simulink model "LLC_26"  (R2022b)
settings: Solver=VariableStepAuto  StartTime=0.0  StopTime=.01  RelTol=1e-3
values from neighbouring files (symbols this model uses):
  tsample_Controller = 20e-6    (= 2e-05)    [LLC_Parameter.m]
  Vref = 500    [LLC_Parameter.m]
undefined symbols (not defined in the file or in its folder): Iref
libraries: fl_lib x137, ee_lib x83, nesl_utility x63, slpidlib x7, slctrlblks x1
(part 1 of 5)
settings Model: Creator=HW-2  LastModifiedBy=Lenovo
settings DebuggingCC: UnconnectedInputMsg=warning  UnconnectedOutputMsg=warning  UnconnectedLineMsg=warning
settings ModelReferenceCC: EnableRefExpFcnMdlSchedulingChecks=on
settings RTWCC: DLArmComputeVersion=19.05

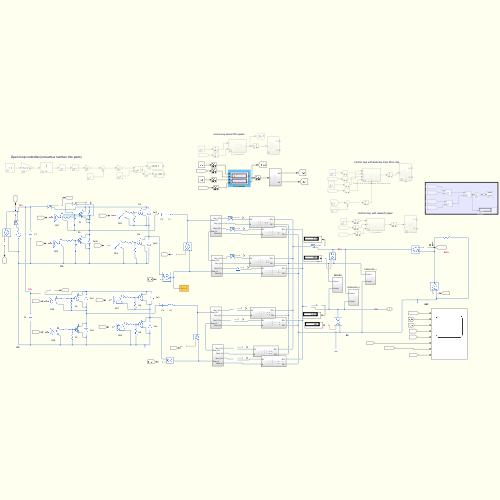
[thumbnail: Simulink's stored preview of the top-level diagram]
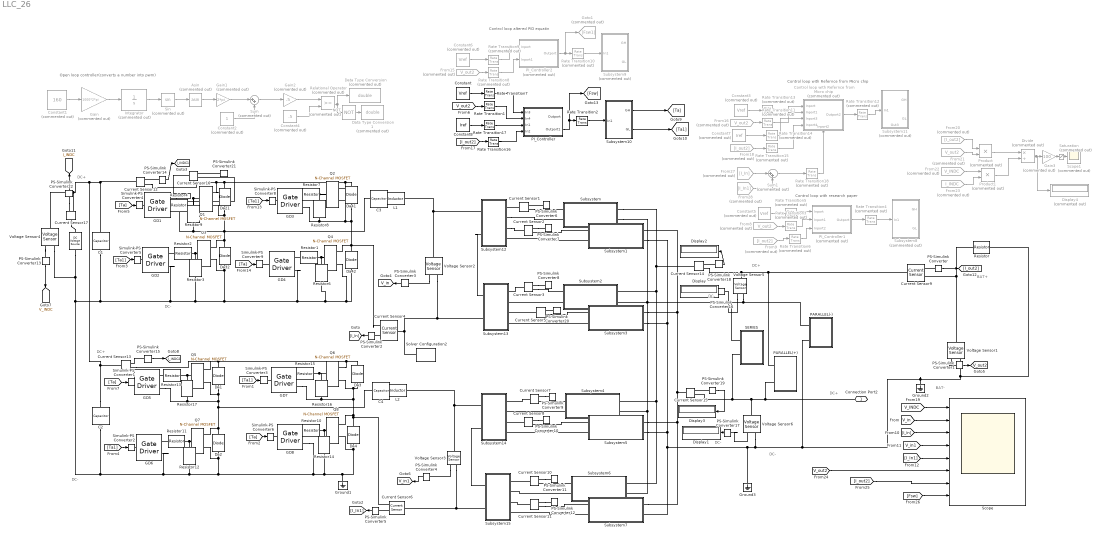
== system LLC_26 ==
  note: Open loop controller(converts a number into pwm)
  note: Control loop altered PID equatin
  note: DC+
  note: Control loop with Refernce from Micro chip
  note: DC-
  note: DC+
  note: Control loop with research paper
  note: BAT-
  note: DC-
  note: DC+
  note: DC-
  note: DC-
  note: DC-
  note: DC+
  note: BAT+
  " " : ee_lib/Additional Components/SPICE Sources/DC Voltage Source  DC=V_INDC V
  Asin : Trigonometry  Commented=on  Operator=asin
  C1 : fl_lib/Electrical/Electrical Elements/Capacitor  c=5e-6 F  r=5e-3 Ohm  g=0 1/Ohm  i_specify=off  i_priority=None  i=0 A  i_nominal_specify=off  i_nominal_unit=A  i_nominal_value=1  v_specify=off  v_priority=None  v=V_INDC V  v_nominal_specify=off  v_nominal_unit=V  v_nominal_value=1  vc_specify=on  vc_priority=High  vc=V_INDC V  vc_nominal_specify=off  vc_nominal_unit=V  vc_nominal_value=1
  C2 : fl_lib/Electrical/Electrical Elements/Capacitor  c=5e-6 F  r=5e-3 Ohm  g=0 1/Ohm  i_specify=off  i_priority=None  i=0 A  i_nominal_specify=off  i_nominal_unit=A  i_nominal_value=1  v_specify=off  v_priority=None  v=V_INDC V  v_nominal_specify=off  v_nominal_unit=V  v_nominal_value=1  vc_specify=on  vc_priority=High  vc=V_INDC V  vc_nominal_specify=off  vc_nominal_unit=V  vc_nominal_value=1
  C3 : fl_lib/Electrical/Electrical Elements/Capacitor  c=Cr F  r=0 Ohm  g=0 1/Ohm  i_specify=off  i_priority=None  i=0 A  i_nominal_specify=off  i_nominal_unit=A  i_nominal_value=1  v_specify=off  v_priority=None  v=0 V  v_nominal_specify=off  v_nominal_unit=V  v_nominal_value=1  vc_specify=off  vc_priority=High  vc=0 V  vc_nominal_specify=off  vc_nominal_unit=V  vc_nominal_value=1
  C4 : fl_lib/Electrical/Electrical Elements/Capacitor  c=Cr F  r=0 Ohm  g=0 1/Ohm  i_specify=off  i_priority=None  i=0 A  i_nominal_specify=off  i_nominal_unit=A  i_nominal_value=1  v_specify=off  v_priority=None  v=0 V  v_nominal_specify=off  v_nominal_unit=V  v_nominal_value=1  vc_specify=off  vc_priority=High  vc=0 V  vc_nominal_specify=off  vc_nominal_unit=V  vc_nominal_value=1
  Constant : Constant  Value=Vref
  Constant1 : Constant  Commented=on  Value=160
  Constant2 : Constant  Commented=on
  Constant3 : Constant  Commented=on  Value=Vref
  Constant4 : Constant  Commented=on  Value=.5
  Constant5 : Constant  Commented=on  Value=Vref
  Constant6 : Constant  Commented=on  Value=Vref
  Constant7 : Constant  Commented=on  Value=Iref
  Constant8 : Constant  Value=Iref
  Control loop with Refernce from Micro chip : Subsystem  Commented=on
      settings: PortSchema="{\"entries\":[{\"content\":{\"sides\":[{\"content\":{\"connectorIds\":[\"In1\",\"In2\",\"In3\",\"In4\"]},\"type\":\"ConnectorPlacement.EquallySpacedRectSide\",\"uuid\":\"8758e69c-c30c-4bdc-ab0d-0d062e0b37b7\"},{\"content\":{\"connectorIds\":[\"Out1\"],\"side\":\"RIGHT\"},\"type\":\"ConnectorPlacement.EquallySpacedRectSide\",\"uuid\":\"dabc2d05-f5c7-433d-b7be-f864c65222bf\"},{\"content\":{\"connectorIds\":[],\"side\":\"TOP\"},\"type\":\"ConnectorPlacement.EquallySpacedRectSide\",\"uuid\":\"e73110cd-836c-4139-8386-715c0e6c244a\"},{\"content\":{\"connectorIds\":[\"In5\"],\"side\":\"BOTTOM\"},\"type\":\"ConnectorPlacement.EquallySpacedRectSide\",\"uuid\":\"c3cb1167-cec3-47ee-be27-ca9bcd7e70cc\"}]},\"type\":\"ConnectorPlacement.EquallySpacedConnector\",\"uuid\":\"6b131b25-3151-447e-9ac8-8b0f0e72c048\"}],\"packageUris\":[\"http://schema.mathworks.com/mf0/Connector/R2020b\"],\"version\":\"1.0\"}"
  Current Sensor{1..17} (17 alike) : fl_lib/Electrical/Electrical Sensors/Current Sensor
  Da{1..4,21,32,41..42} (8 alike) : ee_lib/Semiconductors & Converters/Diode  ModelType=ee.enum.diode.modelType.pwl  TableType=ee.enum.diode.tableType.IfMat  IfMat=[.07, .12, .19, 1.75, 4.24, 7.32, 11.2; .16, .3, .72, 2.14, 4.02, 6.35, 9.12] A  VfMat=[.9, 1.15, 1.25, 1.5, 1.75, 2.17, 2.6, 2.85; .58, .68, .75, 1.1, 1.38, 1.77, 2.27, 2.7] V  TjVec=[25, 125] degC  VfVec=[.5, .7, .9, 1.3, 1.7, 2.1, 2.5] V  IfVec=[.1, .2, .5, 1, 2, 4, 7, 10] A  Vf=Vf V  Ron=Ron Ohm  Goff=1e-8 1/Ohm  prmExp=ee.enum.diode.expParam.useTwo  I12=[.0137, .545] A  V12=[.6, .7] V  RS=0 Ohm  Tmeas=25 degC  IS=1e-12 A  ec=1  I1=0.0137 A  V1=0.6 V  N_series=1  N_parallel=1  Rz=0.3 Ohm  BV=inf V  C_param=ee.enum.diode.capParam.fixed  CJ=0 pF  CJ0=5 pF  Vvec=[.1, 10, 100] V  Cvec=[3.5, 1, .4] pF  VJ=1 V  Mgrad=0.5  FC=0.5  Q_param=ee.enum.diode.recoveryParam.off  iRM=-7.15 A  iF=4 A  didt=-750 A/us  trr_factor=3  trr=115 ns  Qrr=1500 s*uA  Vr=-600 V  Ls=150 nH  Erec=0.03 J  TT=50 ns  tau=100 ns  T_param=ee.enum.diode.temperatureParam.off  Tdevice=25 degC  I1_T2=0.245 A  V1_T2=0.5 V  IS_T2=1.25e-7 A  Tmeas2=125 degC  XTI_param=ee.enum.diode.xtiParam.pn  XTI=3  EG_param=ee.enum.diode.egapParam.material_si  EG=1.11 eV  dBVdT=0 V/K  enable_faults=simscape.enum.onoff.off  fault_action=simscape.enum.assert.action.none  fault_types=ee.enum.diode.faults.open  tau_fault=1e-3 s  IfMat_faulted=[.07, .12, .19, 1.75, 4.24, 7.32, 11.2; .16, .3, .72, 2.14, 4.02, 6.35, 9.12] A  VfMat_faulted=[.9, 1.15, 1.25, 1.5, 1.75, 2.17, 2.6, 2.85; .58, .68, .75, 1.1, 1.38, 1.77, 2.27, 2.7] V  VfVec_faulted=[.5, .7, .9, 1.3, 1.7, 2.1, 2.5] V  IfVec_faulted=[.1, .2, .5, 1, 2, 4, 7, 10] A  Ropen_faulted=1000 Ohm  Gshort_faulted=1000 1/Ohm  Vf_faulted=0.6 V  Ron_faulted=0.3 Ohm  Goff_faulted=1e-8 S  I12_faulted=[.0137, .545] A  V12_faulted=[.6, .7] V  IS_faulted=1e-12 A  ec_faulted=1  I1_faulted=0.0137 A  V1_faulted=0.6 V  RS_faulted=0 Ohm  Rz_faulted=0.3 Ohm  BV_faulted=inf V  Cscale_faulted=100  enable_temporal_fault=simscape.enum.onoff.off  t_fault=inf s  enable_behavioral_fault=simscape.enum.onoff.off  max_permissible_voltage=inf V  n_fail_on_voltage=1  max_permissible_current=inf A  t_fail_on_current=1 s  max_permissible_dVdt=inf V/s  enable_fault_input=simscape.enum.onoff.off  i_specify=off  i_priority=None  i=0 A  i_nominal_specify=off  i_nominal_unit=A  i_nominal_value=1  v_specify=off  v_priority=None  v=0 V  v_nominal_specify=off  v_nominal_unit=V  v_nominal_value=1  v_capacitor_specify=off  v_capacitor_priority=None  v_capacitor=0 V  v_capacitor_nominal_specify=off  v_capacitor_nominal_unit=V  v_capacitor_nominal_value=1  i_diode_specify=off  i_diode_priority=None  i_diode=0 A  i_diode_nominal_specify=off  i_diode_nominal_unit=A  i_diode_nominal_value=1  v_diode_specify=off  v_diode_priority=None  v_diode=0 V  v_diode_nominal_specify=off  v_diode_nominal_unit=V  v_diode_nominal_value=1  i_capacitor_specify=off  i_capacitor_priority=None  i_capacitor=0 A  i_capacitor_nominal_specify=off  i_capacitor_nominal_unit=A  i_capacitor_nominal_value=1  power_dissipated_specify=off  power_dissipated_priority=None  power_dissipated=0 W  power_dissipated_nominal_specify=off  power_dissipated_nominal_unit=W  power_dissipated_nominal_value=1  fidelity_level=ee.enum.diode.fidelity.includeChargeDyn  rec_loss_model=ee.enum.diode.reverseRecoveryModel.fixed  ErecVal=0 J  ErecMat=zeros(2, 3) J  TjrecVec=[298.15, 398.15] K  IfrecVec=[.1, 1, 10] A  VrecVal=10 V  tFilter=1 / 1000 / 100 s  max_permissible_temperature=inf K  t_fail_on_temperature=1 s  thermal_network_parameterization=ee.enum.thermalNetworkTopology.junctionCase  Rth=[0, 10] K/W  Rth_Cauer=[1, 3, 10] K/W  Rth_Foster=[4, 6] K/W  thermal_mass_parameterization=ee.enum.thermalNetwork.timeconstant  thermal_mass=[0, 1] J/K  thermal_mass_Cauer=[.1, .3, 1] J/K  thermal_mass_Foster=[1.5, 3] J/K  thermal_time_constant=[0, 10] s  thermal_time_constant_Cauer=[1, 3, 10] s  thermal_time_constant_Foster=[6, 18] s  thermal_mass_initial_temperatures=[25, 25] degC  thermal_mass_initial_temperatures_Cauer=[25, 25, 25] degC  junction_thermal_mass=0.01 J/K  Tvec_initial_Foster=[25, 25, 25, 25] degC  no_thermal_network=0  junction_temperature_specify=off  junction_temperature_priority=None  junction_temperature=25 degC  junction_temperature_nominal_specify=off  junction_temperature_nominal_unit=degC  junction_temperature_nominal_value=1
  Data Type Conversion : DataTypeConversion  Commented=on  OutDataTypeStr=double  SaturateOnIntegerOverflow=off  RndMeth=Floor
  Data Type Conversion1 : DataTypeConversion  Commented=on  OutDataTypeStr=double  SaturateOnIntegerOverflow=off  RndMeth=Floor
  Display{,1..3} (4 alike) : Display
  Display4 : Display  Commented=on
  Divide : Product  Commented=on  Inputs=*/
  From{8,15..16,21} (4 alike) : From  Commented=on  GotoTag=V_out2  TagVisibility=global
  From18 : From  Commented=on  GotoTag=I_out2
  From20 : From  Commented=on  GotoTag=I_out2
  From22 : From  Commented=on  GotoTag=V_INDC  TagVisibility=global
  From23 : From  Commented=on  GotoTag=I_INDC  TagVisibility=global
  From27 : From  Commented=on  GotoTag=I_In
  From28 : From  Commented=on  GotoTag=I_In1
  From9 : From  Commented=on  GotoTag=I_out2
  GD{1..8} (8 alike) : ee_lib/Semiconductors & Converters/Gate Driver  uHighValue=0.7  uLowValue=0.3  vHigh=18 V  vLow=-3 V  tHigh=50 ns  tLow=50 ns  parameterization=1  rHigh=2 Ohm  rLow=2 Ohm  tRise=20 ns  tFall=20 ns  cLoad=10 nF  enable_faults=0  t_fault=1 s  fault_type=1  ZonTime_specify=off  ZonTime_priority=None  ZonTime=0 s  ZoffTime_specify=off  ZoffTime_priority=None  ZoffTime=0 s  uHigh=2.0 V  uLow=0.8 V
      settings: InternalSimscapePortConfiguration="{\"Bottom\":[],\"Left\":[{\"id\":\"u\",\"label\":\"u\",\"type\":\"input\"}],\"Right\":[{\"id\":\"G\",\"label\":\"G\",\"type\":\"foundation.electrical.electrical\"},{\"id\":\"S\",\"label\":\"S\",\"type\":\"foundation.electrical.electrical\"}],\"Top\":[]}"
  Gain : Gain  Commented=on  Gain=1000*2*pi
  Gain1 : Gain  Commented=on  Gain=2*pi
  Gain2 : Gain  Commented=on  Gain=.5
  Gain3 : Gain  Commented=on  Gain=100
  Goto1 : Goto  Commented=on  GotoTag=Fsw1
  Ground1 : fl_lib/Electrical/Electrical Elements/Electrical Reference
  Ground2 : fl_lib/Electrical/Electrical Elements/Electrical Reference
  Ground3 : fl_lib/Electrical/Electrical Elements/Electrical Reference
  Integrator : Integrator  Commented=on
  L1 : fl_lib/Electrical/Electrical Elements/Inductor  l=Lr H  r=0 Ohm  g=0 1/Ohm  i_specify=off  i_priority=None  i=0 A  i_nominal_specify=off  i_nominal_unit=A  i_nominal_value=1  v_specify=off  v_priority=None  v=0 V  v_nominal_specify=off  v_nominal_unit=V  v_nominal_value=1  i_L_specify=off  i_L_priority=High  i_L=0 A  i_L_nominal_specify=off  i_L_nominal_unit=A  i_L_nominal_value=1
  L2 : fl_lib/Electrical/Electrical Elements/Inductor  l=Lr H  r=0 Ohm  g=0 1/Ohm  i_specify=off  i_priority=None  i=0 A  i_nominal_specify=off  i_nominal_unit=A  i_nominal_value=1  v_specify=off  v_priority=None  v=0 V  v_nominal_specify=off  v_nominal_unit=V  v_nominal_value=1  i_L_specify=off  i_L_priority=High  i_L=0 A  i_L_nominal_specify=off  i_L_nominal_unit=A  i_L_nominal_value=1
  NOT : Logic  Commented=on  Operator=NOT  IconShape=distinctive  AllPortsSameDT=off  OutDataTypeStr=boolean
  PARALLEL(+) : Subsystem
  PARALLEL(-) : Subsystem
  PI_Controller : Subsystem
  PI_Controller1 : Subsystem  Commented=on
  PI_Controller2 : Subsystem  Commented=on
  PS-Simulink Converter{,1..22} (23 alike) : nesl_utility/PS-Simulink Converter  PhysicalDomain=network_engine_domain  SubClassName=ps_output  LeftPortType=input  RightPortType=output  PseudoPeriodic=off  Frequencies=[]  VectorFormat=1-D array  Unit=inherit  AffineConversion=off
  Product : Product  Commented=on
  Product1 : Product  Commented=on
  Q{1,3..8} (7 alike) : ee_lib/Semiconductors & Converters/N-Channel MOSFET  paramTerminal=ee.enum.mosfet.numberOfTerminals.three  parameterization=ee.enum.mosfet.parameterization.datasheet  Beta=5.0 A/V^2  Rds=0.042 Ohm  Id=100 A  Vgs=20 V  Vth=3.8 V  Vth0=2.8 V  lam=0 1/V  gamma_vth=0.5 V^0.50000  phib=0.5 V  Vth1=4 V  Vbs1=-1 V  Vth2=5 V  Vbs2=-2 V  Tmeas=125 degC  Vgs_vec=[-.5, 2, 3, 4, 5] V  Vds_vec=[0, 2, 4, 8, 12, 16, 20] V  Vbs_vec=[0, -4, -6, -12] V  T_vec=[25, 125] degC  Vth_vec=[.4, 1.2, 1.4, 1.45] V  Vth_mat=[.4, .35; 1.2, 1.15; 1.4, 1.35; 1.45, 1.4] V  Ids_mat=[0, 0, 0, 0, 0, 0, 0; 0, .003, .0038, .0043, .0046, .0048, .0049; 0, .0055, .008, .009, .0095, .01, .0101; 0, .0115, .016, .018, .019, .0195, .02; 0, .0152, .0225, .0265, .028, .0295, .03] A  Ids_mat0=[0, 0, 0, 0, 0, 0, 0; 0, .003, .0038, .0043, .0046, .0048, .0049; 0, .0055, .008, .009, .0095, .01, .0101; 0, .0115, .016, .018, .019, .0195, .02; 0, .0152, .0225, .0265, .028, .0295, .03] A  Ids_mat_3D=zeros(5, 7, 2) A  Ids_mat_3D0=zeros(5, 7, 2) A  IV_table_symmetry=ee.enum.mosfet.symmetricNIV.no  RS=1e-3 Ohm  RD=0.1e-3 Ohm  RB=0.001 Ohm  C_param=ee.enum.mosfet.capacitanceParam.fixedciss  C_GS=270 pF  C_GD=80 pF  C_GB=0 pF  C_DS=0 pF  C_iss=2320 pF  C_rss=9 pF  C_oss=111 pF  C_iss_vec=[720, 700, 590, 470, 390, 310] pF  C_rss_vec=[450, 400, 300, 190, 95, 55] pF  C_oss_vec=[900, 810, 690, 420, 270, 170] pF  C_GS_vec=[270, 300, 290, 280, 295, 255] pF  C_GD_vec=[450, 400, 300, 190, 95, 55] pF  C_GB_vec=[270, 300, 290, 280, 295, 255] pF  C_Vgs_vec=0 V  C_DS_vec=[450, 410, 390, 230, 175, 115] pF  C_Vds_vec=[.1, .3, 1, 3, 10, 30] V  V_GS_for_cap_data=0 V  charge_linearity_param=ee.enum.mosfet.cgdLinearity.constant  C_OX=200 pF  V_C_OX=-0.5 V  charge_linearity_param_vgb=ee.enum.mosfet.cgbLinearity.instantly  charge_linearity_param_with_vgb=ee.enum.mosfet.cgbLinearityWithSeparateCgb.instantly  Di_param=ee.enum.mosfet.diodeParam.no  IsDiode=0 A  Vbi=0.6 V  n=1  Cj0Diode=0 pF  TT=50e-9 s  Tmeas_dio=25 degC  TableTypeNoT=ee.enum.mosfet.tableType.IfMat  TableType=ee.enum.diode.tableType.IfMat  IfVec=[.07, .12, .19, 1.75, 4.24, 7.32, 11.2] A  IfMat=[.07, .12, .19, 1.75, 4.24, 7.32, 11.2; .16, .3, .72, 2.14, 4.02, 6.35, 9.12] A  VfVecV=[.9, 1.15, 1.25, 1.5, 1.75, 2.17, 2.6, 2.85] V  VfMatV=[.9, 1.15, 1.25, 1.5, 1.75, 2.17, 2.6, 2.85; .58, .68, .75, 1.1, 1.38, 1.77, 2.27, 2.7] V  TjVec=[25, 125] degC  VfVec=[.5, .7, .9, 1.3, 1.7, 2.1, 2.5] V  IfVecV=[.1, .2, .5, 1, 2, 4, 7, 10] A  prmDatasheet=ee.enum.temperatureParameterization.none  prmEquCoeff=ee.enum.temperatureParameterization.none  dVth_dT=-6 mV/K  dVth0_dT=-6 mV/K  Rds_T2=0.037 Ohm  BEXDatasheet=-1.5  BEXEquCoeff=-1.5  etaisDatasheet=3  etaisEquCoeff=3  Tmeas2=125 degC  etaisTabulated=3  TdeviceDatasheet=25 degC  TdeviceEquCoeff=25 degC  TdeviceTabulated=25 degC  enable_faults=simscape.enum.onoff.off  fault_trigger=ee.enum.faults.faultTrigger.temporal  t_fault=inf s  max_permissible_Vgs=inf V  max_permissible_Vds=inf V  max_permissible_Vdb=inf V  max_permissible_Ids=inf A  t_fail_on_Ids=1 s  max_permissible_Idiode=inf A  t_fail_on_Idiode=1 s  max_permissible_dVdt=inf V/s  tau_fault=1e-3 s  fault_types=ee.enum.mosfet.faults.open  fault_types_4T=ee.enum.mosfet.faultsFourTerminals.open  RG_open=1e6 Ohm  RD_open=1000 Ohm  RS_open=1000 Ohm  RB_open=1000 Ohm  GDS_short=1000 1/Ohm  GDB_short=1000 1/Ohm  GSB_short=1000 1/Ohm  location_GOS=0  G_GOS=1000 1/Ohm  D_GOS=ee.enum.include.no  Is_GOS=0 A  Vbi_GOS=0.6 V  n_GOS=1  Cj0_GOS=0 pF  TT_GOS=50e-9 s  Beta_scale=100  dVth_faulted=0 V  lam_faulted=0 1/V  gamma_scale=100  dPhib_faulted=0 V  Vgs_vec_faulted=[-.5, 2, 3, 4, 5] V  Vds_vec_faulted=[0, 2, 4, 8, 12, 16, 20] V  Vbs_vec_faulted=[0, -4, -6, -12] V  Vth_vec_faulted=[.4, 1.2, 1.4, 1.45] V  Vth_mat_faulted=[.4, .35; 1.2, 1.15; 1.4, 1.35; 1.45, 1.4] V  Ids_mat_faulted=[0, 0, 0, 0, 0, 0, 0; 0, .003, .0038, .0043, .0046, .0048, .0049; 0, .0055, .008, .009, .0095, .01, .0101; 0, .0115, .016, .018, .019, .0195, .02; 0, .0152, .0225, .0265, .028, .0295, .03] A  Ids_mat0_faulted=[0, 0, 0, 0, 0, 0, 0; 0, .003, .0038, .0043, .0046, .0048, .0049; 0, .0055, .008, .009, .0095, .01, .0101; 0, .0115, .016, .018, .019, .0195, .02; 0, .0152, .0225, .0265, .028, .0295, .03] A  Ids_mat_3D_faulted=zeros(5, 7, 2) A  Ids_mat_3D0_faulted=zeros(5, 7, 2) A  RS_faulted=0.0001 Ohm  RD_faulted=0.01 Ohm  RB_faulted=0.001 Ohm  IsDiode_faulted=0 A  Vbi_faulted=0.6 V  n_faulted=1  Cj0Diode_scale=100  TT_faulted=50e-9 s  IfVec_faulted=[.07, .12, .19, 1.75, 4.24, 7.32, 11.2] A  IfMat_faulted=[.07, .12, .19, 1.75, 4.24, 7.32, 11.2; .16, .3, .72, 2.14, 4.02, 6.35, 9.12] A  VfVecV_faulted=[.9, 1.15, 1.25, 1.5, 1.75, 2.17, 2.6, 2.85] V  VfMatV_faulted=[.9, 1.15, 1.25, 1.5, 1.75, 2.17, 2.6, 2.85; .58, .68, .75, 1.1, 1.38, 1.77, 2.27, 2.7] V  VfVec_faulted=[.5, .7, .9, 1.3, 1.7, 2.1, 2.5] V  IfVecV_faulted=[.1, .2, .5, 1, 2, 4, 7, 10] A  C_GS_scale=100  C_GD_scale=100  C_GB_scale=100  C_DS_scale=100  C_OX_scale=100  V_C_OX_faulted=-0.5 V  C_iss_vec_faulted=[720, 700, 590, 470, 390, 310] pF  C_rss_vec_faulted=[450, 400, 300, 190, 95, 55] pF  C_oss_vec_faulted=[900, 810, 690, 420, 270, 170] pF  C_GS_vec_faulted=[270, 300, 290, 280, 295, 255] pF  C_GD_vec_faulted=[450, 400, 300, 190, 95, 55] pF  C_GB_vec_faulted=[270, 300, 290, 280, 295, 255] pF  C_Vgs_vec_faulted=0 V  C_DS_vec_faulted=[450, 410, 390, 230, 175, 115] pF  C_Vds_vec_faulted=[.1, .3, 1, 3, 10, 30] V  V_GS_for_cap_data_faulted=0 V  i_g_specify=off  i_g_priority=None  i_g=0 A  i_g_nominal_specify=off  i_g_nominal_unit=A  i_g_nominal_value=1  i_d_specify=off  i_d_priority=None  i_d=0 A  i_d_nominal_specify=off  i_d_nominal_unit=A  i_d_nominal_value=1  i_b_specify=off  i_b_priority=None  i_b=0 A  i_b_nominal_specify=off  i_b_nominal_unit=A  i_b_nominal_value=1  voltage_gs_specify=off  voltage_gs_priority=None  voltage_gs=0 V  voltage_gs_nominal_specify=off  voltage_gs_nominal_unit=V  voltage_gs_nominal_value=1  voltage_ds_specify=off  voltage_ds_priority=None  voltage_ds=0 V  voltage_ds_nominal_specify=off  voltage_ds_nominal_unit=V  voltage_ds_nominal_value=1  voltage_bs_specify=off  voltage_bs_priority=None  voltage_bs=0 V  voltage_bs_nominal_specify=off  voltage_bs_nominal_unit=V  voltage_bs_nominal_value=1  v_Cgs_specify=off  v_Cgs_priority=High  v_Cgs=0 V  v_Cgs_nominal_specify=off  v_Cgs_nominal_unit=V  v_Cgs_nominal_value=1  v_Cds_specify=off  v_Cds_priority=High  v_Cds=0 V  v_Cds_nominal_specify=off  v_Cds_nominal_unit=V  v_Cds_nominal_value=1  v_Cbs_specify=off  v_Cbs_priority=High  v_Cbs=0 V  v_Cbs_nominal_specify=off  v_Cbs_nominal_unit=V  v_Cbs_nominal_value=1  thermal_network_parameterization=ee.enum.thermalNetworkTopology.junctionCase  Rth=[0, 10] K/W  Rth_Cauer=[1, 3, 10] K/W  Rth_Foster=[4, 6] K/W  thermal_mass_parameterization=ee.enum.thermalNetwork.timeconstant  thermal_mass=[0, 1] J/K  thermal_mass_Cauer=[.1, .3, 1] J/K  thermal_mass_Foster=[1.5, 3] J/K  thermal_time_constant=[0, 10] s  thermal_time_constant_Cauer=[1, 3, 10] s  thermal_time_constant_Foster=[6, 18] s  thermal_mass_initial_temperatures=[25, 25] degC  thermal_mass_initial_temperatures_Cauer=[25, 25, 25] degC  Tvec_initial_Foster=[25, 25, 25, 25] degC  max_permissible_temperature=inf K  t_fail_on_temperature=1 s  betaref=18 A/V^2  Vfbref=-1.1 V  gamma=3.5 V^(1/2)  phib2ref=1 V  thesatref=0.4 1/V  alpha=0  Vp=5e-2 V  thesrref=0 1/V  m=8  Tref=25 degC  Rsref=2e-3 Ohm  Rdref=0.17 Ohm  Rgref=8.4 Ohm  Rbref=2e-3 Ohm  Cox=1500 pF  Cgso=100 pF  Cgdo=14 pF  Isref=5.2e-13 A  Cj0=480 pF  Tprm=1  etabet=1.3  Stvfb=5e-4 V/K  Stphib=-8.5e-4 V/K  etasat=1.04  etasr=0.65  etar=0.95  etais=3  Tsim=25 degC  Ig_specify=off  Ig_priority=None  Ig=0 A  Ig_nominal_specify=off  Ig_nominal_unit=A  Ig_nominal_value=1  Ids_specify=off  Ids_priority=None  Ids=0 A  Ids_nominal_specify=off  Ids_nominal_unit=A  Ids_nominal_value=1  Ib_specify=off  Ib_priority=None  Ib=0 A  Ib_nominal_specify=off  Ib_nominal_unit=A  Ib_nominal_value=1  V_gs_specify=off  V_gs_priority=None  V_gs=0 V  V_gs_nominal_specify=off  V_gs_nominal_unit=V  V_gs_nominal_value=1  V_ds_specify=off  V_ds_priority=None  V_ds=0 V  V_ds_nominal_specify=off  V_ds_nominal_unit=V  V_ds_nominal_value=1  V_bs_specify=off  V_bs_priority=None  V_bs=0 V  V_bs_nominal_specify=off  V_bs_nominal_unit=V  V_bs_nominal_value=1  QGoverCox_specify=off  QGoverCox_priority=None  QGoverCox=0 V  QGoverCox_nominal_specify=off  QGoverCox_nominal_unit=V  QGoverCox_nominal_value=1  QDoverCox_specify=off  QDoverCox_priority=None  QDoverCox=0 V  QDoverCox_nominal_specify=off  QDoverCox_nominal_unit=V  QDoverCox_nominal_value=1  QBoverCox_specify=off  QBoverCox_priority=None  QBoverCox=0 V  QBoverCox_nominal_specify=off  QBoverCox_nominal_unit=V  QBoverCox_nominal_value=1  T0=[25, 25] degC  T0_Cauer=[25, 25, 25] degC
  "Q2 " : ee_lib/Semiconductors & Converters/N-Channel MOSFET  paramTerminal=ee.enum.mosfet.numberOfTerminals.three  parameterization=ee.enum.mosfet.parameterization.datasheet  Beta=5.0 A/V^2  Rds=0.042 Ohm  Id=100 A  Vgs=20 V  Vth=3.8 V  Vth0=2.8 V  lam=0 1/V  gamma_vth=0.5 V^0.50000  phib=0.5 V  Vth1=4 V  Vbs1=-1 V  Vth2=5 V  Vbs2=-2 V  Tmeas=125 degC  Vgs_vec=[-.5, 2, 3, 4, 5] V  Vds_vec=[0, 2, 4, 8, 12, 16, 20] V  Vbs_vec=[0, -4, -6, -12] V  T_vec=[25, 125] degC  Vth_vec=[.4, 1.2, 1.4, 1.45] V  Vth_mat=[.4, .35; 1.2, 1.15; 1.4, 1.35; 1.45, 1.4] V  Ids_mat=[0, 0, 0, 0, 0, 0, 0; 0, .003, .0038, .0043, .0046, .0048, .0049; 0, .0055, .008, .009, .0095, .01, .0101; 0, .0115, .016, .018, .019, .0195, .02; 0, .0152, .0225, .0265, .028, .0295, .03] A  Ids_mat0=[0, 0, 0, 0, 0, 0, 0; 0, .003, .0038, .0043, .0046, .0048, .0049; 0, .0055, .008, .009, .0095, .01, .0101; 0, .0115, .016, .018, .019, .0195, .02; 0, .0152, .0225, .0265, .028, .0295, .03] A  Ids_mat_3D=zeros(5, 7, 2) A  Ids_mat_3D0=zeros(5, 7, 2) A  IV_table_symmetry=ee.enum.mosfet.symmetricNIV.no  RS=1e-3 Ohm  RD=0.1e-3 Ohm  RB=0.001 Ohm  C_param=ee.enum.mosfet.capacitanceParam.fixedciss  C_GS=270 pF  C_GD=80 pF  C_GB=0 pF  C_DS=0 pF  C_iss=2320 pF  C_rss=9 pF  C_oss=111 pF  C_iss_vec=[720, 700, 590, 470, 390, 310] pF  C_rss_vec=[450, 400, 300, 190, 95, 55] pF  C_oss_vec=[900, 810, 690, 420, 270, 170] pF  C_GS_vec=[270, 300, 290, 280, 295, 255] pF  C_GD_vec=[450, 400, 300, 190, 95, 55] pF  C_GB_vec=[270, 300, 290, 280, 295, 255] pF  C_Vgs_vec=0 V  C_DS_vec=[450, 410, 390, 230, 175, 115] pF  C_Vds_vec=[.1, .3, 1, 3, 10, 30] V  V_GS_for_cap_data=0 V  charge_linearity_param=ee.enum.mosfet.cgdLinearity.constant  C_OX=200 pF  V_C_OX=-0.5 V  charge_linearity_param_vgb=ee.enum.mosfet.cgbLinearity.instantly  charge_linearity_param_with_vgb=ee.enum.mosfet.cgbLinearityWithSeparateCgb.instantly  Di_param=ee.enum.mosfet.diodeParam.no  IsDiode=0 A  Vbi=0.6 V  n=1  Cj0Diode=0 pF  TT=50e-9 s  Tmeas_dio=25 degC  TableTypeNoT=ee.enum.mosfet.tableType.IfMat  TableType=ee.enum.diode.tableType.IfMat  IfVec=[.07, .12, .19, 1.75, 4.24, 7.32, 11.2] A  IfMat=[.07, .12, .19, 1.75, 4.24, 7.32, 11.2; .16, .3, .72, 2.14, 4.02, 6.35, 9.12] A  VfVecV=[.9, 1.15, 1.25, 1.5, 1.75, 2.17, 2.6, 2.85] V  VfMatV=[.9, 1.15, 1.25, 1.5, 1.75, 2.17, 2.6, 2.85; .58, .68, .75, 1.1, 1.38, 1.77, 2.27, 2.7] V  TjVec=[25, 125] degC  VfVec=[.5, .7, .9, 1.3, 1.7, 2.1, 2.5] V  IfVecV=[.1, .2, .5, 1, 2, 4, 7, 10] A  prmDatasheet=ee.enum.temperatureParameterization.none  prmEquCoeff=ee.enum.temperatureParameterization.none  dVth_dT=-6 mV/K  dVth0_dT=-6 mV/K  Rds_T2=0.037 Ohm  BEXDatasheet=-1.5  BEXEquCoeff=-1.5  etaisDatasheet=3  etaisEquCoeff=3  Tmeas2=125 degC  etaisTabulated=3  TdeviceDatasheet=25 degC  TdeviceEquCoeff=25 degC  TdeviceTabulated=25 degC  enable_faults=simscape.enum.onoff.off  fault_trigger=ee.enum.faults.faultTrigger.temporal  t_fault=inf s  max_permissible_Vgs=inf V  max_permissible_Vds=inf V  max_permissible_Vdb=inf V  max_permissible_Ids=inf A  t_fail_on_Ids=1 s  max_permissible_Idiode=inf A  t_fail_on_Idiode=1 s  max_permissible_dVdt=inf V/s  tau_fault=1e-3 s  fault_types=ee.enum.mosfet.faults.open  fault_types_4T=ee.enum.mosfet.faultsFourTerminals.open  RG_open=1e6 Ohm  RD_open=1000 Ohm  RS_open=1000 Ohm  RB_open=1000 Ohm  GDS_short=1000 1/Ohm  GDB_short=1000 1/Ohm  GSB_short=1000 1/Ohm  location_GOS=0  G_GOS=1000 1/Ohm  D_GOS=ee.enum.include.no  Is_GOS=0 A  Vbi_GOS=0.6 V  n_GOS=1  Cj0_GOS=0 pF  TT_GOS=50e-9 s  Beta_scale=100  dVth_faulted=0 V  lam_faulted=0 1/V  gamma_scale=100  dPhib_faulted=0 V  Vgs_vec_faulted=[-.5, 2, 3, 4, 5] V  Vds_vec_faulted=[0, 2, 4, 8, 12, 16, 20] V  Vbs_vec_faulted=[0, -4, -6, -12] V  Vth_vec_faulted=[.4, 1.2, 1.4, 1.45] V  Vth_mat_faulted=[.4, .35; 1.2, 1.15; 1.4, 1.35; 1.45, 1.4] V  Ids_mat_faulted=[0, 0, 0, 0, 0, 0, 0; 0, .003, .0038, .0043, .0046, .0048, .0049; 0, .0055, .008, .009, .0095, .01, .0101; 0, .0115, .016, .018, .019, .0195, .02; 0, .0152, .0225, .0265, .028, .0295, .03] A  Ids_mat0_faulted=[0, 0, 0, 0, 0, 0, 0; 0, .003, .0038, .0043, .0046, .0048, .0049; 0, .0055, .008, .009, .0095, .01, .0101; 0, .0115, .016, .018, .019, .0195, .02; 0, .0152, .0225, .0265, .028, .0295, .03] A  Ids_mat_3D_faulted=zeros(5, 7, 2) A  Ids_mat_3D0_faulted=zeros(5, 7, 2) A  RS_faulted=0.0001 Ohm  RD_faulted=0.01 Ohm  RB_faulted=0.001 Ohm  IsDiode_faulted=0 A  Vbi_faulted=0.6 V  n_faulted=1  Cj0Diode_scale=100  TT_faulted=50e-9 s  IfVec_faulted=[.07, .12, .19, 1.75, 4.24, 7.32, 11.2] A  IfMat_faulted=[.07, .12, .19, 1.75, 4.24, 7.32, 11.2; .16, .3, .72, 2.14, 4.02, 6.35, 9.12] A  VfVecV_faulted=[.9, 1.15, 1.25, 1.5, 1.75, 2.17, 2.6, 2.85] V  VfMatV_faulted=[.9, 1.15, 1.25, 1.5, 1.75, 2.17, 2.6, 2.85; .58, .68, .75, 1.1, 1.38, 1.77, 2.27, 2.7] V  VfVec_faulted=[.5, .7, .9, 1.3, 1.7, 2.1, 2.5] V  IfVecV_faulted=[.1, .2, .5, 1, 2, 4, 7, 10] A  C_GS_scale=100  C_GD_scale=100  C_GB_scale=100  C_DS_scale=100  C_OX_scale=100  V_C_OX_faulted=-0.5 V  C_iss_vec_faulted=[720, 700, 590, 470, 390, 310] pF  C_rss_vec_faulted=[450, 400, 300, 190, 95, 55] pF  C_oss_vec_faulted=[900, 810, 690, 420, 270, 170] pF  C_GS_vec_faulted=[270, 300, 290, 280, 295, 255] pF  C_GD_vec_faulted=[450, 400, 300, 190, 95, 55] pF  C_GB_vec_faulted=[270, 300, 290, 280, 295, 255] pF  C_Vgs_vec_faulted=0 V  C_DS_vec_faulted=[450, 410, 390, 230, 175, 115] pF  C_Vds_vec_faulted=[.1, .3, 1, 3, 10, 30] V  V_GS_for_cap_data_faulted=0 V  i_g_specify=off  i_g_priority=None  i_g=0 A  i_g_nominal_specify=off  i_g_nominal_unit=A  i_g_nominal_value=1  i_d_specify=off  i_d_priority=None  i_d=0 A  i_d_nominal_specify=off  i_d_nominal_unit=A  i_d_nominal_value=1  i_b_specify=off  i_b_priority=None  i_b=0 A  i_b_nominal_specify=off  i_b_nominal_unit=A  i_b_nominal_value=1  voltage_gs_specify=off  voltage_gs_priority=None  voltage_gs=0 V  voltage_gs_nominal_specify=off  voltage_gs_nominal_unit=V  voltage_gs_nominal_value=1  voltage_ds_specify=off  voltage_ds_priority=None  voltage_ds=0 V  voltage_ds_nominal_specify=off  voltage_ds_nominal_unit=V  voltage_ds_nominal_value=1  voltage_bs_specify=off  voltage_bs_priority=None  voltage_bs=0 V  voltage_bs_nominal_specify=off  voltage_bs_nominal_unit=V  voltage_bs_nominal_value=1  v_Cgs_specify=off  v_Cgs_priority=High  v_Cgs=0 V  v_Cgs_nominal_specify=off  v_Cgs_nominal_unit=V  v_Cgs_nominal_value=1  v_Cds_specify=off  v_Cds_priority=High  v_Cds=0 V  v_Cds_nominal_specify=off  v_Cds_nominal_unit=V  v_Cds_nominal_value=1  v_Cbs_specify=off  v_Cbs_priority=High  v_Cbs=0 V  v_Cbs_nominal_specify=off  v_Cbs_nominal_unit=V  v_Cbs_nominal_value=1  thermal_network_parameterization=ee.enum.thermalNetworkTopology.junctionCase  Rth=[0, 10] K/W  Rth_Cauer=[1, 3, 10] K/W  Rth_Foster=[4, 6] K/W  thermal_mass_parameterization=ee.enum.thermalNetwork.timeconstant  thermal_mass=[0, 1] J/K  thermal_mass_Cauer=[.1, .3, 1] J/K  thermal_mass_Foster=[1.5, 3] J/K  thermal_time_constant=[0, 10] s  thermal_time_constant_Cauer=[1, 3, 10] s  thermal_time_constant_Foster=[6, 18] s  thermal_mass_initial_temperatures=[25, 25] degC  thermal_mass_initial_temperatures_Cauer=[25, 25, 25] degC  Tvec_initial_Foster=[25, 25, 25, 25] degC  max_permissible_temperature=inf K  t_fail_on_temperature=1 s  betaref=18 A/V^2  Vfbref=-1.1 V  gamma=3.5 V^(1/2)  phib2ref=1 V  thesatref=0.4 1/V  alpha=0  Vp=5e-2 V  thesrref=0 1/V  m=8  Tref=25 degC  Rsref=2e-3 Ohm  Rdref=0.17 Ohm  Rgref=8.4 Ohm  Rbref=2e-3 Ohm  Cox=1500 pF  Cgso=100 pF  Cgdo=14 pF  Isref=5.2e-13 A  Cj0=480 pF  Tprm=1  etabet=1.3  Stvfb=5e-4 V/K  Stphib=-8.5e-4 V/K  etasat=1.04  etasr=0.65  etar=0.95  etais=3  Tsim=25 degC  Ig_specify=off  Ig_priority=None  Ig=0 A  Ig_nominal_specify=off  Ig_nominal_unit=A  Ig_nominal_value=1  Ids_specify=off  Ids_priority=None  Ids=0 A  Ids_nominal_specify=off  Ids_nominal_unit=A  Ids_nominal_value=1  Ib_specify=off  Ib_priority=None  Ib=0 A  Ib_nominal_specify=off  Ib_nominal_unit=A  Ib_nominal_value=1  V_gs_specify=off  V_gs_priority=None  V_gs=0 V  V_gs_nominal_specify=off  V_gs_nominal_unit=V  V_gs_nominal_value=1  V_ds_specify=off  V_ds_priority=None  V_ds=0 V  V_ds_nominal_specify=off  V_ds_nominal_unit=V  V_ds_nominal_value=1  V_bs_specify=off  V_bs_priority=None  V_bs=0 V  V_bs_nominal_specify=off  V_bs_nominal_unit=V  V_bs_nominal_value=1  QGoverCox_specify=off  QGoverCox_priority=None  QGoverCox=0 V  QGoverCox_nominal_specify=off  QGoverCox_nominal_unit=V  QGoverCox_nominal_value=1  QDoverCox_specify=off  QDoverCox_priority=None  QDoverCox=0 V  QDoverCox_nominal_specify=off  QDoverCox_nominal_unit=V  QDoverCox_nominal_value=1  QBoverCox_specify=off  QBoverCox_priority=None  QBoverCox=0 V  QBoverCox_nominal_specify=off  QBoverCox_nominal_unit=V  QBoverCox_nominal_value=1  T0=[25, 25] degC  T0_Cauer=[25, 25, 25] degC
  Rate Transition{1,7,16..17} (4 alike) : RateTransition  OutPortSampleTime=tsample_Controller
  Rate Transition10 : RateTransition  Commented=on
  Rate Transition{3,5..6,8..9,11,13..15,18} (10 alike) : RateTransition  Commented=on  OutPortSampleTime=tsample_Controller
  Rate Transition12 : RateTransition  Commented=on
  Rate Transition2 : RateTransition
  Rate Transition4 : RateTransition  Commented=on
  Relational Operator : RelationalOperator  Commented=on  OutDataTypeStr=boolean  RndMeth=Simplest  InputSameDT=off
  Resistor : ee_lib/Passive/Resistor  R=1000 Ohm  enable_R_tol=0  R_tol=5  tol_distribution=1  nSigma=4  enable_operating_limits=0  operating_limit_action=2  max_working_voltage=100 V  power_rating=1 W  enable_faults=0  fault_action=1  R_faulted=inf Ohm  enable_temporal_fault=0  t_fault=1 s  enable_behavioral_fault=0  max_permissible_current=1 A  t_fail_on_current=1 s  noise_mode=0  sample_time=1e-3 s  repeatability=1  auto_seed=4169120344  user_seed=0  Tdevice=25 degC  power_derating_T1=70 degC  power_derating_T2=155 degC  operating_temperature_range_vec=[-50, 150] degC  alpha=3.93e-3 1/K  Tmeas=25 degC  thermal_mass=100 J/K  temperature_specify=off  temperature_priority=High  temperature=298.15 K  temperature_nominal_specify=off  temperature_nominal_unit=K  temperature_nominal_value=1
  Resistor{1..2,4,7,10..11,13,15} (8 alike) : fl_lib/Electrical/Electrical Elements/Resistor  R=10 Ohm  i_specify=off  i_priority=None  i=0 A  i_nominal_specify=off  i_nominal_unit=A  i_nominal_value=1  v_specify=off  v_priority=None  v=0 V  v_nominal_specify=off  v_nominal_unit=V  v_nominal_value=1
  Resistor{3,6,8..9,12,14,16..17} (8 alike) : fl_lib/Electrical/Electrical Elements/Resistor  R=10 kOhm  i_specify=off  i_priority=None  i=0 A  i_nominal_specify=off  i_nominal_unit=A  i_nominal_value=1  v_specify=off  v_priority=None  v=0 V  v_nominal_specify=off  v_nominal_unit=V  v_nominal_value=1
  SERIES : Subsystem
  Saturation : Saturate  Commented=on  UpperLimit=100  LowerLimit=0
  Scope : Scope  NumInputPorts=8
  Scope1 : Scope  Commented=on
  Simulink-PS Converter{1..6,8..9} (8 alike) : nesl_utility/Simulink-PS Converter  PhysicalDomain=network_engine_domain  SubClassName=ps_input  LeftPortType=input  RightPortType=output  PseudoPeriodic=off  Frequencies=[]  NoiseDistribution=none  NoiseParameters=[]  Unit=1  AffineConversion=off  FilteringAndDerivatives=provide  SimscapeFilterOrder=1  InputFilterTimeConstant=0.001  UdotUserProvided=0
  Sin : Trigonometry  Commented=on
  Solver Configuration2 : nesl_utility/Solver Configuration  PhysicalDomain=network_engine_domain  SubClassName=solver  LeftPortType=input  RightPortType=generic  Tones=[]  Harmonics=[]  SimulateNoise=off  Profile=off  UseLocalSampling=off  EnableSwitchedLinearOptims=on  FrequencyDomain=off  UseCCode=off  RelTol=0.001  AbsTol=1e-06  MinStep=1e-09  ToWorkspace=off  RevertToSquareIcSolve=off  NumHomotopyIterations=100  PhasorMode=off  PhasorModeNumHarmonics=1  ConsistencySolver=NEWTON_FTOL  IndexReductionMethod=DerivativeReplacement  DoDC=off  ResidualTolerance=1e-09  ConsistencyTolSource=GLOBAL  ConsistencyAbsTol=0.001  ConsistencyRelTol=0.001  ConsistencyTolFactor=0.001  UseLocalSolver=on  LocalSolverChoice=NE_BACKWARD_EULER_ADVANCER  ResolveIndetEquations=on  FunctionEvalNumThread=1  LocalSolverSampleTime=1e-7  DoFixedCost=off  MaxNonlinIter=4  MaxModeIter=2  ComputeImpulses=off  ImpulseIterations=2  LinearAlgebra=auto  LinearAlgebraNumThread=0  EquationFormulation=NE_TIME_EF  DelaysMemoryBudget=1024  AutomaticFiltering=on  FilteringTimeConstant=0.001  PartitionStorageMethod=AS_NEEDED  PartitionMemoryBudget=1024  PartitionMethod=FAST
  Subsystem : Subsystem
  Subsystem1 : Subsystem
  Subsystem10 : Subsystem
  Subsystem11 : Subsystem  Commented=on
      settings: PortSchema="{\"entries\":[{\"content\":{\"sides\":[{\"content\":{\"connectorIds\":[\"In1\"]},\"type\":\"ConnectorPlacement.EquallySpacedRectSide\",\"uuid\":\"c53c7d2c-8aa3-4151-82be-c10e714e6679\"},{\"content\":{\"connectorIds\":[\"Out1\",\"Out2\"],\"side\":\"RIGHT\"},\"type\":\"ConnectorPlacement.EquallySpacedRectSide\",\"uuid\":\"a42cc241-e860-4882-947f-0eda612eaf4a\"},{\"content\":{\"connectorIds\":[],\"side\":\"TOP\"},\"type\":\"ConnectorPlacement.EquallySpacedRectSide\",\"uuid\":\"2bd5491d-7597-4a9e-b246-390268707e73\"},{\"content\":{\"connectorIds\":[\"Out3\"],\"side\":\"BOTTOM\"},\"type\":\"ConnectorPlacement.EquallySpacedRectSide\",\"uuid\":\"b6ed39f1-a382-41e3-860b-700ff50b0320\"}]},\"type\":\"ConnectorPlacement.EquallySpacedConnector\",\"uuid\":\"917fb526-c419-4f1f-a687-cdd96705cb3d\"}],\"packageUris\":[\"http://schema.mathworks.com/mf0/Connector/R2020b\"],\"version\":\"1.0\"}"
  Subsystem12 : Subsystem
  Subsystem13 : Subsystem
  Subsystem14 : Subsystem
  Subsystem15 : Subsystem
  Subsystem2 : Subsystem
  Subsystem3 : Subsystem
  Subsystem4 : Subsystem
  Subsystem5 : Subsystem
  Subsystem6 : Subsystem
  Subsystem7 : Subsystem
  Subsystem8 : Subsystem  Commented=on
  Subsystem9 : Subsystem  Commented=on
  Sum : Sum  Commented=on  Inputs=|++
  Sum1 : Sum  Commented=on  Inputs=|++
  Voltage Sensor{1..6} (6 alike) : fl_lib/Electrical/Electrical Sensors/Voltage Sensor
  Connection Port2 : PMIOPort  Side=Left
  tag scope: I_INDC1=global, I_INDC2=global, I_INDC=global, V_INDC=global, V_in1=global, V_in=global, V_out2=global
  wires:
  Gain3/1 -> Saturation/1
  PS-Simulink Converter15/1 -> [I_INDC2]
  Saturation/1 -> Scope1/1
  Control loop with Refernce from Micro chip/1(Outport2) -> Rate Transition12/1
  From22/1 -> Product1/1
  Constant3/1 -> Rate Transition13/1
  From21/1 -> Product/2
  Product1/1 -> Divide/2
  Constant8/1 -> Rate Transition17/1
  From23/1 -> Product1/2
  Rate Transition8/1 -> PI_Controller2/2(Inport1)
  PS-Simulink Converter22/1 -> [I_INDC]
  [V_in1] -> Scope/4
  Rate Transition17/1 -> PI_Controller/3(In1)
  Divide/1 -> Display4/1, Gain3/1
  PS-Simulink Converter1/1 -> [V_out2]
  From9/1 -> Rate Transition6/1
  [V_INDC] -> Scope/1
  PS-Simulink Converter/1 -> [I_out2]
  Constant7/1 -> Rate Transition14/1
  PS-Simulink Converter16/1 -> Display/1
  Rate Transition14/1 -> Control loop with Refernce from Micro chip/3(Inport3)
  Rate Transition15/1 -> Control loop with Refernce from Micro chip/4(Inport4)
  From18/1 -> Rate Transition15/1
  [Ta1] -> Simulink-PS Converter8/1
  PS-Simulink Converter14/1 -> [I_INDC1]
  Rate Transition13/1 -> Control loop with Refernce from Micro chip/1(Inport)
  PS-Simulink Converter5/1 -> [I_In1]
  [I_out2] -> Rate Transition16/1
  Constant6/1 -> Rate Transition9/1
  Rate Transition3/1 -> PI_Controller1/2(Inport1)
  PI_Controller1/1(Outport) -> Rate Transition4/1
  Rate Transition11/1 -> Control loop with Refernce from Micro chip/2(Inport1)
  Constant2/1 -> Sum/2
  Rate Transition6/1 -> PI_Controller1/3(Inport2)
  Rate Transition2/1 -> Subsystem10/1(In1)
  PS-Simulink Converter17/1 -> Display1/1
  PS-Simulink Converter19/1 -> Display3/1
  Constant5/1 -> Rate Transition5/1
  [Ta] -> Simulink-PS Converter6/1
  Constant/1 -> Rate Transition7/1
  Rate Transition5/1 -> PI_Controller1/1(Inport)
  Rate Transition4/1 -> Subsystem8/1(In1)
  [V_in] -> Scope/2
  PS-Simulink Converter18/1 -> Display2/1
  [I_In] -> Scope/3
  Gain/1 -> Integrator/1
  Asin/1 -> Gain1/1
  Gain2/1 -> Relational Operator/1
  From8/1 -> Rate Transition3/1
  Constant1/1 -> Gain/1
  NOT/1 -> Data Type Conversion1/1
  [Ta1] -> Simulink-PS Converter2/1
  PI_Controller2/1(Outport) -> Goto1/1, Rate Transition10/1
  [V_out2] -> Scope/6
  [Ta] -> Simulink-PS Converter9/1
  Rate Transition7/1 -> PI_Controller/1(In3)
  Sin/1 -> Asin/1
  PS-Simulink Converter4/1 -> [V_in1]
  From20/1 -> Product/1
  Rate Transition1/1 -> PI_Controller/2(In4)
  PS-Simulink Converter3/1 -> [V_in]
  [Ta] -> Simulink-PS Converter1/1
  [I_In1] -> Scope/5
  From16/1 -> Rate Transition11/1
  [Ta] -> Simulink-PS Converter4/1
  PS-Simulink Converter13/1 -> [V_INDC]
  Sum/1 -> Gain2/1
  [Fsw] -> Scope/8
  Rate Transition16/1 -> PI_Controller/4(In2)
  Integrator/1 -> Sin/1
  [I_out2] -> Scope/7
  Gain1/1 -> Sum/1
  Rate Transition10/1 -> Subsystem9/1(In1)
  [Ta1] -> Simulink-PS Converter3/1
  Constant4/1 -> Relational Operator/2
  PS-Simulink Converter2/1 -> [I_In]
  Relational Operator/1 -> Data Type Conversion/1, NOT/1
  [Ta1] -> Simulink-PS Converter5/1
  Rate Transition12/1 -> Subsystem11/1(In1)
  Rate Transition9/1 -> PI_Controller2/1(Inport)
  From15/1 -> Rate Transition8/1
  [V_out2] -> Rate Transition1/1
  Product/1 -> Divide/1
  Sum1/1 -> Rate Transition18/1
  From27/1 -> Sum1/1
  From28/1 -> Sum1/2
  Rate Transition18/1 -> Control loop with Refernce from Micro chip/5(Inport2)
  Subsystem10/2(GL) -> [Ta1]
  Subsystem10/1(GH) -> [Ta]
  PI_Controller/2(Outport1) -> [Fsw], Rate Transition2/1
  connections:
  Subsystem6/RConn2 -- Subsystem4/RConn2 -- PARALLEL(-)/RConn1 -- Voltage Sensor5/RConn2 -- SERIES/RConn1 -- Subsystem/RConn2 -- Subsystem2/RConn2
  Voltage Sensor2/RConn2 -- Subsystem13/LConn2 -- Current Sensor4/LConn1 -- Solver Configuration2/RConn1
  Voltage Sensor3/LConn1 -- Subsystem14/LConn1 -- L2/RConn1
  Resistor10/RConn1 -- Q8/LConn1 -- Resistor14/LConn1
  L1/RConn1 -- Voltage Sensor2/LConn1 -- Subsystem12/LConn1
  Current Sensor15/LConn1 -- Subsystem1/RConn1 -- Subsystem3/RConn1 -- Subsystem7/RConn1 -- Subsystem5/RConn1
  Q6/LConn1 -- Resistor16/LConn1 -- Resistor15/RConn1
  "Q2 "/RConn1 -- Da41/RConn1 -- Current Sensor12/RConn2 -- Q1/RConn1 -- Da21/RConn1
  Resistor4/RConn1 -- Resistor9/LConn1 -- Q1/LConn1
  Subsystem6/RConn1 -- Subsystem4/RConn1 -- Subsystem/RConn1 -- Current Sensor14/LConn1 -- Subsystem2/RConn1
  Resistor1/RConn1 -- Q4/LConn1 -- Resistor6/LConn1
  Voltage Sensor3/RConn2 -- Subsystem15/LConn2 -- Current Sensor6/LConn1
  Da41/LConn1 -- Q4/RConn1 -- Current Sensor4/RConn2 -- Da42/RConn1 -- Resistor8/RConn1 -- GD3/RConn2 -- "Q2 "/RConn2
  Da3/LConn1 -- Resistor16/RConn1 -- GD7/RConn2 -- Current Sensor6/RConn2 -- Da4/RConn1 -- Q8/RConn1 -- Q6/RConn2
  Current Sensor9/RConn2 -- Resistor/LConn1 -- Voltage Sensor1/LConn1
  Resistor2/RConn1 -- Resistor3/LConn1 -- Q3/LConn1
  Da1/LConn1 -- Q5/RConn2 -- GD5/RConn2 -- Resistor17/RConn1 -- Q7/RConn1 -- Da2/RConn1 -- C4/LConn1
  Q1/RConn2 -- Da21/LConn1 -- Da32/RConn1 -- Q3/RConn1 -- GD1/RConn2 -- Resistor9/RConn1 -- C3/LConn1
  GD8/RConn2 -- Ground1/LConn1 -- Da4/LConn1 -- Q8/RConn2 -- Resistor14/RConn1 -- Da2/LConn1 -- Q7/RConn2 -- Resistor12/RConn1 -- GD6/RConn2 -- C2/RConn1 -- Voltage Sensor4/RConn2 -- " "/RConn1 -- C1/RConn1 -- GD2/RConn2 -- Da32/LConn1 -- Q3/RConn2 -- GD4/RConn2 -- Q4/RConn2 -- Da42/LConn1 -- Resistor6/RConn1 -- Resistor3/RConn1
  Resistor7/RConn1 -- Resistor8/LConn1 -- "Q2 "/LConn1
  Resistor13/RConn1 -- Resistor17/LConn1 -- Q5/LConn1
  C2/LConn1 -- Voltage Sensor4/LConn1 -- Current Sensor17/RConn2 -- C1/LConn1 -- Current Sensor12/LConn1 -- Current Sensor13/LConn1
  PARALLEL(-)/RConn2 -- Subsystem5/RConn2 -- Subsystem1/RConn2 -- Subsystem3/RConn2 -- Subsystem7/RConn2 -- Ground3/LConn1 -- Voltage Sensor6/RConn2 -- Resistor/RConn1 -- Voltage Sensor1/RConn2 -- Ground2/LConn1
  Resistor11/RConn1 -- Resistor12/LConn1 -- Q7/LConn1
  PARALLEL(+)/RConn2 -- Voltage Sensor6/LConn1 -- SERIES/RConn2 -- Current Sensor15/RConn2 -- Connection Port2/RConn1
  Voltage Sensor5/LConn1 -- PARALLEL(+)/RConn1 -- Current Sensor9/LConn1 -- Current Sensor14/RConn2
  Q5/RConn1 -- Da3/RConn1 -- Q6/RConn1 -- Current Sensor13/RConn2 -- Da1/RConn1
  Current Sensor10/RConn1 -- PS-Simulink Converter11/LConn1
  Current Sensor11/RConn1 -- PS-Simulink Converter12/LConn1
  PS-Simulink Converter20/LConn1 -- Current Sensor5/RConn1
  PS-Simulink Converter13/LConn1 -- Voltage Sensor4/RConn1
  Current Sensor1/LConn1 -- Subsystem12/RConn1
  Current Sensor10/RConn2 -- Subsystem6/LConn1
  PS-Simulink Converter19/LConn1 -- Current Sensor15/RConn1
  Subsystem14/LConn2 -- Subsystem15/LConn1
  PS-Simulink Converter15/LConn1 -- Current Sensor13/RConn1
  Current Sensor8/LConn1 -- Subsystem14/RConn3
  Current Sensor7/RConn1 -- PS-Simulink Converter9/LConn1
  Subsystem7/LConn2 -- Subsystem15/RConn4
  Current Sensor17/LConn1 -- " "/LConn1
  Current Sensor5/LConn1 -- Subsystem13/RConn3
  GD1/RConn1 -- Current Sensor16/LConn1
  GD4/RConn1 -- Resistor1/LConn1
  Voltage Sensor5/RConn1 -- PS-Simulink Converter16/LConn1
  Resistor4/LConn1 -- Current Sensor16/RConn2
  GD2/RConn1 -- Resistor2/LConn1
  Voltage Sensor2/RConn1 -- PS-Simulink Converter3/LConn1
  Current Sensor3/RConn2 -- Subsystem2/LConn1
  GD5/LConn1 -- Simulink-PS Converter1/RConn1
  GD7/RConn1 -- Resistor15/LConn1
  GD8/LConn1 -- Simulink-PS Converter6/RConn1
  Subsystem5/LConn1 -- Current Sensor8/RConn2
  PS-Simulink Converter/LConn1 -- Current Sensor9/RConn1
  GD5/RConn1 -- Resistor13/LConn1
  Current Sensor7/RConn2 -- Subsystem4/LConn1
  Current Sensor3/LConn1 -- Subsystem13/RConn1
  Current Sensor8/RConn1 -- PS-Simulink Converter10/LConn1
  Current Sensor2/RConn2 -- Subsystem1/LConn1
  Subsystem2/LConn2 -- Subsystem13/RConn2
  Subsystem5/LConn2 -- Subsystem14/RConn4
  GD4/LConn1 -- Simulink-PS Converter9/RConn1
  GD6/RConn1 -- Resistor11/LConn1
  Simulink-PS Converter4/RConn1 -- GD1/LConn1
  Subsystem6/LConn2 -- Subsystem15/RConn2
  L2/LConn1 -- C4/RConn1
  GD3/LConn1 -- Simulink-PS Converter8/RConn1
  GD7/LConn1 -- Simulink-PS Converter3/RConn1
  Current Sensor11/LConn1 -- Subsystem15/RConn3
  PS-Simulink Converter17/LConn1 -- Voltage Sensor6/RConn1
  Subsystem1/LConn2 -- Subsystem12/RConn4
  PS-Simulink Converter2/LConn1 -- Current Sensor4/RConn1
  Subsystem4/LConn2 -- Subsystem14/RConn2
  Current Sensor3/RConn1 -- PS-Simulink Converter8/LConn1
  GD6/LConn1 -- Simulink-PS Converter2/RConn1
  Subsystem12/LConn2 -- Subsystem13/LConn1
  PS-Simulink Converter1/LConn1 -- Voltage Sensor1/RConn1
  Voltage Sensor3/RConn1 -- PS-Simulink Converter4/LConn1
  Subsystem12/RConn3 -- Current Sensor2/LConn1
  PS-Simulink Converter22/LConn1 -- Current Sensor17/RConn1
  Current Sensor2/RConn1 -- PS-Simulink Converter7/LConn1
  Current Sensor1/RConn2 -- Subsystem/LConn1
  Current Sensor7/LConn1 -- Subsystem14/RConn1
  Current Sensor6/RConn1 -- PS-Simulink Converter5/LConn1
  PS-Simulink Converter6/LConn1 -- Current Sensor1/RConn1
  GD3/RConn1 -- Resistor7/LConn1
  PS-Simulink Converter18/LConn1 -- Current Sensor14/RConn1
  GD2/LConn1 -- Simulink-PS Converter5/RConn1
  L1/LConn1 -- C3/RConn1
  Current Sensor5/RConn2 -- Subsystem3/LConn1
  Current Sensor11/RConn2 -- Subsystem7/LConn1
  PS-Simulink Converter14/LConn1 -- Current Sensor12/RConn1
  Subsystem3/LConn2 -- Subsystem13/RConn4
  GD8/RConn1 -- Resistor10/LConn1
  PS-Simulink Converter21/LConn1 -- Current Sensor16/RConn1
  Current Sensor10/LConn1 -- Subsystem15/RConn1
  Subsystem12/RConn2 -- Subsystem/LConn2
